simulink model "H175_Stage_01_Anode_Cathode"  (R2023a)
settings: Solver=VariableStepAuto  StartTime=0.0  StopTime=500  RelTol=1e-3
values from neighbouring files (symbols this model uses):
  anode_tube_D = 0.01    [All_Properties.mat]    (also in anode_subsystem_parameters.m; environment_parameters.m)
  D = 0.01    [All_Properties.mat]    (also in anode_subsystem_parameters.m)
  densityHydrogen = 0.0899    [All_Properties.mat]    (also in Valve_Init.m; anode_subsystem_parameters.m)
  Fischer_EMTC120K_supplier_mdot_TLU = [33.385172 57.11265182 82.35238332 173.9183787 230.2050798 50.1655574 86.1774137 122.96585 210.0188714 258.8737112 70.20710678 115.3896052 ... (25 elements, 5x5)]    [All_Properties.mat]    (also in cathode_subsystem_parameters.m = [33.385172 50.1655574 70.20710678 87.4902972 105.3161257)
  Fischer_EMTC120K_supplier_pr_TLU = [2.452176848 3.067593046 4.01020547 5.11549365 6.10066015 2.450765612 3.07166407 4.0616557 5.112468546 6.108742034 2.432340262 3.033516574 ... (25 elements, 5x5)]    [All_Properties.mat]    (also in cathode_subsystem_parameters.m = [2.452176848 2.450765612 2.432340262 2.407245766 2.37067916)
  Kv_VL6112 = 0.8    [All_Properties.mat]    (also in anode_subsystem_parameters.m)
  N2_T = [-56.55 -50 -40 -30 -20 -10 -5 -4 -3 -2 -1 0 ... (52 elements, 1x52)]    [All_Properties.mat]    (also in anode_subsystem_parameters.m = [-56.55 -50 -40 -30 -20 -10 -5 -4 -3 -2 -1 0 1 2 3 4 5 10 20; environment_parameters.m = [-56.55, -50:10:-10, -5:1:5, 10:10:350]; stack_model_harness_parameters.m = [-56.55, -50:10:-10, -5:1:5, 10:10:350])
  p_range = 0.005    [All_Properties.mat]    (also in anode_subsystem_parameters.m)
  r_max = 0.2    [All_Properties.mat]    (also in anode_subsystem_parameters.m)
  r_min = 0.0001    [All_Properties.mat]    (also in anode_subsystem_parameters.m)
  responseTimeValve = 0.013    [All_Properties.mat]    (also in anode_subsystem_parameters.m)
undefined symbols (not defined in the file or in its folder): sigbuilder_block
libraries: fl_lib x168, nesl_utility x116, SimscapeFluids_lib x8, slpidlib x5, simulink x1
(part 6 of 8)

== system H175_Stage_01_Anode_Cathode/Plant Model H175-Cathode-S1/LT-Cooling ==
  Convective Heat Transfer1 : fl_lib/Thermal/Thermal Elements/Convective Heat Transfer  thermal_type=foundation.enum.constant_variable.constant  area=10.8 m^2  heat_tr_coeff=3465 W/(m^2 * K)  min_heat_tr_coeff=1e-3 W/(K*m^2)  T_specify=off  T_priority=None  T=0 K  T_nominal_specify=off  T_nominal_unit=K  T_nominal_value=1  Q_specify=off  Q_priority=None  Q=0 W  Q_nominal_specify=off  Q_nominal_unit=W  Q_nominal_value=1
  Convective Heat Transfer2 : fl_lib/Thermal/Thermal Elements/Convective Heat Transfer  thermal_type=foundation.enum.constant_variable.constant  area=10.8 m^2  heat_tr_coeff=447*4 W/(m^2 * K)  min_heat_tr_coeff=1e-3 W/(K*m^2)  T_specify=off  T_priority=None  T=0 K  T_nominal_specify=off  T_nominal_unit=K  T_nominal_value=1  Q_specify=off  Q_priority=None  Q=0 W  Q_nominal_specify=off  Q_nominal_unit=W  Q_nominal_value=1
  Coolant Tank1 : Subsystem  Tag=PublishSubsystem  mask(Coolant Tank){A=100, x_init=.25}
      mask prompts: A "Tank area (m^2)"; x_init "Initial coolant level (m)"
      mask help: This subsystem models an expansion tank for the coolant system.
  Environment Temperature4 : fl_lib/Thermal/Thermal Sources/Temperature Source  temperature=20 degC
  Glysantin G20 : SimscapeFluids_lib/Thermal Liquid/Utilities/Thermal Liquid Properties (TL)  fluid_list=fluids.thermal_liquid.utilities.enum.thermal_liquid_fluid_list.ethylene_glycol  concentration_param_EG=fluids.thermal_liquid.utilities.enum.thermal_liquid_concentration.volume_fraction  concentration_param_PG=fluids.thermal_liquid.utilities.enum.thermal_liquid_concentration.volume_fraction  c_mass_SW=3.5e-3  c_mass_EG=0.1  c_mass_PG=0.1  c_mass_GL=0.1  c_vol_EG=0.5  c_vol_PG=0.1  beta_const_EG=2.1791 GPa  beta_const_PG=2.1791 GPa  beta_const_GL=2.1791 GPa  p_min_EG=0.01 MPa  p_min_PG=0.01 MPa  p_min_GL=0.01 MPa  p_max_EG=50 MPa  p_max_PG=50 MPa  p_max_GL=50 MPa  p_atm=1 bar  properties_range_check=simscape.enum.assert.action.error
  Pipe (TL)1 : fl_lib/Thermal Liquid/Elements/Pipe (TL)  length=1 m  area=10.8 m^2  Dh=0.1 m  length_add=10 m  roughness=15e-6 m  Re_lam=2000  Re_tur=4000  shape_factor=64  Nu_lam=133.3  dynamic_compressibility=simscape.enum.onoff.on  inertia=simscape.enum.onoff.off  p0=0.101325 MPa  T0=293.15 K  mdot0=0 kg/s
  Pump1 : fl_lib/Thermal Liquid/Sources/Controlled Mass Flow Rate Source (TL)  power_spec=foundation.enum.power_spec.isentropic  area=.002 m^2
      settings: InternalSimscapePortConfiguration="{\"Bottom\":[],\"Left\":[{\"id\":\"A\",\"label\":\"A\",\"type\":\"foundation.thermal_liquid.thermal_liquid\"},{\"id\":\"M\",\"label\":\"M\",\"type\":\"input\"}],\"Right\":[{\"id\":\"B\",\"label\":\"B\",\"type\":\"foundation.thermal_liquid.thermal_liquid\"}],\"Top\":[]}"
  Radiator1 : fl_lib/Thermal Liquid/Elements/Pipe (TL)  length=1 m  area=10.8 m^2  Dh=.1 m  length_add=1 m  roughness=15e-6 m  Re_lam=2000  Re_tur=4000  shape_factor=64  Nu_lam=500  dynamic_compressibility=simscape.enum.onoff.on  inertia=simscape.enum.onoff.off  p0=.103 MPa  T0=20 degC  mdot0=0 kg/s
  Thermal Mass1 : fl_lib/Thermal/Thermal Elements/Thermal Mass  mass_type=foundation.enum.constant_variable.constant  mass=5 kg  sp_heat=447 J/(K*kg)  mass_min=1e-6 kg  num_ports=foundation.enum.numPorts2.two  m_specify=off  m_priority=High  m=1 kg  m_nominal_specify=off  m_nominal_unit=kg  m_nominal_value=1  T_specify=off  T_priority=High  T=300 K  T_nominal_specify=off  T_nominal_unit=K  T_nominal_value=1  Q_specify=off  Q_priority=None  Q=0 W  Q_nominal_specify=off  Q_nominal_unit=W  Q_nominal_value=1
      settings: InternalSimscapePortConfiguration="{\"Bottom\":[],\"Left\":[{\"id\":\"M\",\"label\":\"\",\"type\":\"foundation.thermal.thermal\"}],\"Right\":[{\"id\":\"N\",\"label\":\"\",\"type\":\"foundation.thermal.thermal\"}],\"Top\":[]}"
  Thermal Mass2 : fl_lib/Thermal/Thermal Elements/Thermal Mass  mass_type=foundation.enum.constant_variable.constant  mass=1 kg  sp_heat=910 J/kg/K  mass_min=1e-6 kg  num_ports=foundation.enum.numPorts2.one  m_specify=off  m_priority=High  m=1 kg  m_nominal_specify=off  m_nominal_unit=kg  m_nominal_value=1  T_specify=on  T_priority=High  T=20 degC  T_nominal_specify=off  T_nominal_unit=K  T_nominal_value=1  Q_specify=off  Q_priority=None  Q=0 W  Q_nominal_specify=off  Q_nominal_unit=W  Q_nominal_value=1
  Conn1 : PMIOPort  Side=Left
  Conn2 : PMIOPort  Port=2  Side=Right
  connections:
  Thermal Mass1/RConn1 -- Pipe (TL)1/LConn2
  Radiator1/LConn1 -- Pipe (TL)1/RConn1
  Convective Heat Transfer1/LConn1 -- Radiator1/LConn2
  Pipe (TL)1/LConn1 -- Glysantin G20/RConn1 -- Pump1/RConn1
  Coolant Tank1/RConn1 -- Pump1/LConn1 -- Radiator1/RConn1
  Conn1/RConn1 -- Pump1/LConn2
  Thermal Mass1/LConn1 -- Convective Heat Transfer2/RConn1
  Convective Heat Transfer1/RConn1 -- Thermal Mass2/LConn1 -- Environment Temperature4/LConn1
  Conn2/RConn1 -- Convective Heat Transfer2/LConn1

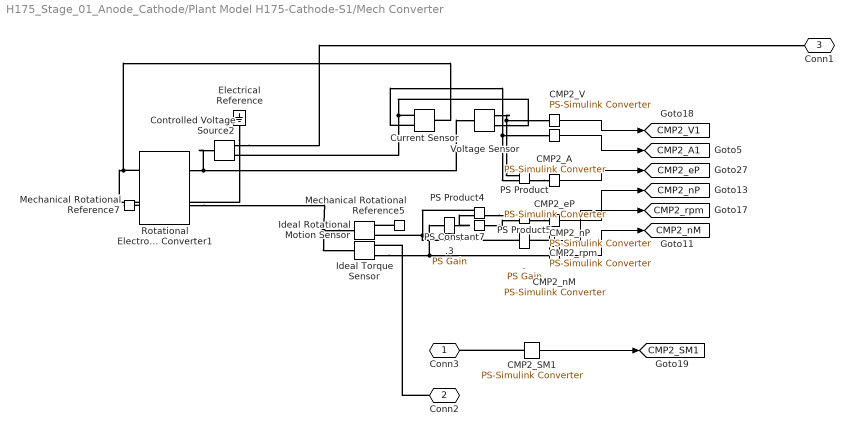
== system H175_Stage_01_Anode_Cathode/Plant Model H175-Cathode-S1/Mech Converter ==
  . : fl_lib/Physical Signals/Functions/PS Gain  gain=1/(0.1047198*1000)
  .3 : fl_lib/Physical Signals/Functions/PS Gain  gain=1/(0.1047198*60)
  CMP2_A : nesl_utility/PS-Simulink Converter  PhysicalDomain=network_engine_domain  SubClassName=ps_output  LeftPortType=input  RightPortType=output  PseudoPeriodic=off  Frequencies=[]  VectorFormat=inherit  Unit=inherit  AffineConversion=off
  CMP2_SM1 : nesl_utility/PS-Simulink Converter  PhysicalDomain=network_engine_domain  SubClassName=ps_output  LeftPortType=input  RightPortType=output  PseudoPeriodic=off  Frequencies=[]  VectorFormat=inherit  Unit=inherit  AffineConversion=off
  CMP2_V : nesl_utility/PS-Simulink Converter  PhysicalDomain=network_engine_domain  SubClassName=ps_output  LeftPortType=input  RightPortType=output  PseudoPeriodic=off  Frequencies=[]  VectorFormat=inherit  Unit=inherit  AffineConversion=off
  CMP2_eP : nesl_utility/PS-Simulink Converter  PhysicalDomain=network_engine_domain  SubClassName=ps_output  LeftPortType=input  RightPortType=output  PseudoPeriodic=off  Frequencies=[]  VectorFormat=inherit  Unit=inherit  AffineConversion=off
  CMP2_nM : nesl_utility/PS-Simulink Converter  PhysicalDomain=network_engine_domain  SubClassName=ps_output  LeftPortType=input  RightPortType=output  PseudoPeriodic=off  Frequencies=[]  VectorFormat=1-D array  Unit=inherit  AffineConversion=off
  CMP2_nP : nesl_utility/PS-Simulink Converter  PhysicalDomain=network_engine_domain  SubClassName=ps_output  LeftPortType=input  RightPortType=output  PseudoPeriodic=off  Frequencies=[]  VectorFormat=inherit  Unit=inherit  AffineConversion=off
  CMP2_rpm : nesl_utility/PS-Simulink Converter  PhysicalDomain=network_engine_domain  SubClassName=ps_output  LeftPortType=input  RightPortType=output  PseudoPeriodic=off  Frequencies=[]  VectorFormat=inherit  Unit=inherit  AffineConversion=off
  Controlled Voltage Source2 : fl_lib/Electrical/Electrical Sources/Controlled Voltage Source
  Current Sensor : fl_lib/Electrical/Electrical Sensors/Current Sensor
  Electrical Reference : fl_lib/Electrical/Electrical Elements/Electrical Reference
  Ideal Rotational Motion Sensor : fl_lib/Mechanical/Mechanical Sensors/Ideal Rotational Motion Sensor  reference=foundation.enum.MeasurementReference.difference  acceleration_port=false  velocity_port=true  position_port=false  wrap_angle=false  offset=0 rad
      settings: InternalSimscapePortConfiguration="{\"Bottom\":[],\"Left\":[{\"id\":\"R\",\"label\":\"R\",\"type\":\"foundation.mechanical.rotational.rotational\"}],\"Right\":[{\"id\":\"C\",\"label\":\"C\",\"type\":\"foundation.mechanical.rotational.rotational\"},{\"id\":\"W\",\"label\":\"W\",\"type\":\"output\"}],\"Top\":[]}"
  Ideal Torque Sensor : fl_lib/Mechanical/Mechanical Sensors/Ideal Torque Sensor
  Mechanical Rotational Reference5 : fl_lib/Mechanical/Rotational Elements/Mechanical Rotational Reference
  Mechanical Rotational Reference7 : fl_lib/Mechanical/Rotational Elements/Mechanical Rotational Reference
  PS Constant7 : fl_lib/Physical Signals/Sources/PS Constant  constant=2*pi
  PS Product : fl_lib/Physical Signals/Functions/PS Product
  PS Product4 : fl_lib/Physical Signals/Functions/PS Product
  PS Product5 : fl_lib/Physical Signals/Functions/PS Product
  Rotational Electromechanical Converter1 : fl_lib/Electrical/Electrical Elements/Rotational Electromechanical Converter  K=0.00409090909090909090909090909091 V/rpm  i_specify=off  i_priority=None  i=0 A  i_nominal_specify=off  i_nominal_unit=A  i_nominal_value=1  v_specify=off  v_priority=None  v=50 V  v_nominal_specify=off  v_nominal_unit=V  v_nominal_value=1  t_specify=off  t_priority=None  t=0 N*m  t_nominal_specify=off  t_nominal_unit=N*m  t_nominal_value=1  w_specify=off  w_priority=None  w=0 rad/s  w_nominal_specify=off  w_nominal_unit=rad/s  w_nominal_value=1
  Voltage Sensor : fl_lib/Electrical/Electrical Sensors/Voltage Sensor
  Conn3 : PMIOPort  Side=Left
  Conn2 : PMIOPort  Port=2  Side=Left
  Conn1 : PMIOPort  Port=3  Side=Right
  tag scope: CMP2_A1=global, CMP2_SM1=global, CMP2_V1=global, CMP2_eP=global, CMP2_nM=global, CMP2_nP=global, CMP2_rpm=global
  wires:
  CMP2_eP/1 -> [CMP2_eP]
  CMP2_V/1 -> [CMP2_V1]
  CMP2_A/1 -> [CMP2_A1]
  CMP2_nM/1 -> [CMP2_nM]
  CMP2_rpm/1 -> [CMP2_rpm]
  CMP2_nP/1 -> [CMP2_nP]
  CMP2_SM1/1 -> [CMP2_SM1]
  connections:
  CMP2_rpm/LConn1 -- ./RConn1
  PS Constant7/RConn1 -- PS Product5/LConn2
  Rotational Electromechanical Converter1/RConn2 -- Mechanical Rotational Reference7/LConn1
  Controlled Voltage Source2/LConn1 -- Voltage Sensor/LConn1 -- Rotational Electromechanical Converter1/LConn1
  Electrical Reference/LConn1 -- Current Sensor/LConn1 -- Rotational Electromechanical Converter1/RConn1
  Current Sensor/RConn1 -- PS Product/LConn1 -- CMP2_A/LConn1
  Controlled Voltage Source2/RConn1 -- Conn1/RConn1
  Ideal Rotational Motion Sensor/LConn1 -- Rotational Electromechanical Converter1/LConn2 -- Ideal Torque Sensor/LConn1
  Current Sensor/RConn2 -- Voltage Sensor/RConn2 -- Controlled Voltage Source2/RConn2
  PS Product/RConn1 -- CMP2_eP/LConn1
  .3/RConn1 -- PS Product4/LConn2
  PS Product4/RConn1 -- PS Product5/LConn1
  Ideal Torque Sensor/RConn2 -- CMP2_nM/LConn1 -- .3/LConn1
  PS Product5/RConn1 -- CMP2_nP/LConn1
  Voltage Sensor/RConn1 -- PS Product/LConn2 -- CMP2_V/LConn1
  ./LConn1 -- PS Product4/LConn1 -- Ideal Rotational Motion Sensor/RConn2
  Mechanical Rotational Reference5/LConn1 -- Ideal Rotational Motion Sensor/RConn1
  Conn2/RConn1 -- Ideal Torque Sensor/RConn1
  CMP2_SM1/LConn1 -- Conn3/RConn1

== system H175_Stage_01_Anode_Cathode/Plant Model H175-Cathode-S1/S1 ==
  Absolute Reference (G) : fl_lib/Gas/Elements/Absolute Reference (G)
      settings: InternalSimscapePortConfiguration="{\"Bottom\":[],\"Left\":[{\"id\":\"A\",\"label\":\"\",\"type\":\"foundation.gas.gas\"}],\"Right\":[],\"Top\":[]}"
  Bus Creator : BusCreator  Inputs=3
  Mass & Energy Flow Rate Sensor (G) : fl_lib/Gas/Sensors/Flow Rate Sensor (G)  mass_flow_measure=true  volumetric_flow_measure=false  volumetric_flow_conditions=foundation.enum.volumetric_flow_conditions.actual  p_std=0.101325 MPa  T_std=20 degC  energy_flow_measure=true
      settings: InternalSimscapePortConfiguration="{\"Bottom\":[{\"id\":\"PHI\",\"label\":\"φ\",\"type\":\"output\"}],\"Left\":[{\"id\":\"A\",\"label\":\"A\",\"type\":\"foundation.gas.gas\"}],\"Right\":[{\"id\":\"B\",\"label\":\"B\",\"type\":\"foundation.gas.gas\"},{\"id\":\"M\",\"label\":\"M\",\"type\":\"output\"}],\"Top\":[]}"
  Pressure & Temperature Sensor (G)4 : fl_lib/Gas/Sensors/Pressure & Temperature Sensor (G)  reference=foundation.enum.MeasurementReference.difference  pressure=true  pressure_spec=foundation.enum.PressureMeasementSpec.Absolute  temperature=true
      settings: InternalSimscapePortConfiguration="{\"Bottom\":[{\"id\":\"T\",\"label\":\"T\",\"type\":\"output\"}],\"Left\":[{\"id\":\"A\",\"label\":\"A\",\"type\":\"foundation.gas.gas\"}],\"Right\":[{\"id\":\"B\",\"label\":\"B\",\"type\":\"foundation.gas.gas\"},{\"id\":\"P\",\"label\":\"P\",\"type\":\"output\"}],\"Top\":[]}"
  aPres_S1 : nesl_utility/PS-Simulink Converter  PhysicalDomain=network_engine_domain  SubClassName=ps_output  LeftPortType=input  RightPortType=output  PseudoPeriodic=off  Frequencies=[]  VectorFormat=inherit  Unit=inherit  AffineConversion=off
  aTemp_S1 : nesl_utility/PS-Simulink Converter  PhysicalDomain=network_engine_domain  SubClassName=ps_output  LeftPortType=input  RightPortType=output  PseudoPeriodic=off  Frequencies=[]  VectorFormat=inherit  Unit=degC  AffineConversion=off
  aTemp_S2 : nesl_utility/PS-Simulink Converter  PhysicalDomain=network_engine_domain  SubClassName=ps_output  LeftPortType=input  RightPortType=output  PseudoPeriodic=off  Frequencies=[]  VectorFormat=inherit  Unit=inherit  AffineConversion=off
  Conn1 : PMIOPort  Side=Left
  Conn2 : PMIOPort  Port=2  Side=Right
  tag scope: S1=global
  wires:
  aTemp_S1/1 -> Bus Creator/2  "aTemp_S1"
  aPres_S1/1 -> Bus Creator/1  "aPres_S1"
  aTemp_S2/1 -> Bus Creator/3  "mFlow_S1"
  Bus Creator/1 -> [S1]
  connections:
  Absolute Reference (G)/LConn1 -- Pressure & Temperature Sensor (G)4/RConn1
  aPres_S1/LConn1 -- Pressure & Temperature Sensor (G)4/RConn2
  aTemp_S1/LConn1 -- Pressure & Temperature Sensor (G)4/RConn3
  Pressure & Temperature Sensor (G)4/LConn1 -- Mass & Energy Flow Rate Sensor (G)/LConn1 -- Conn1/RConn1
  Mass & Energy Flow Rate Sensor (G)/RConn2 -- aTemp_S2/LConn1
  Mass & Energy Flow Rate Sensor (G)/RConn1 -- Conn2/RConn1

== system H175_Stage_01_Anode_Cathode/Plant Model H175-Cathode-S1/S2 ==
  Absolute Reference (G) : fl_lib/Gas/Elements/Absolute Reference (G)
      settings: InternalSimscapePortConfiguration="{\"Bottom\":[],\"Left\":[{\"id\":\"A\",\"label\":\"\",\"type\":\"foundation.gas.gas\"}],\"Right\":[],\"Top\":[]}"
  Bus Creator : BusCreator  Inputs=3
  Mass & Energy Flow Rate Sensor (G) : fl_lib/Gas/Sensors/Flow Rate Sensor (G)  mass_flow_measure=true  volumetric_flow_measure=false  volumetric_flow_conditions=foundation.enum.volumetric_flow_conditions.actual  p_std=0.101325 MPa  T_std=20 degC  energy_flow_measure=true
      settings: InternalSimscapePortConfiguration="{\"Bottom\":[{\"id\":\"PHI\",\"label\":\"φ\",\"type\":\"output\"}],\"Left\":[{\"id\":\"A\",\"label\":\"A\",\"type\":\"foundation.gas.gas\"}],\"Right\":[{\"id\":\"B\",\"label\":\"B\",\"type\":\"foundation.gas.gas\"},{\"id\":\"M\",\"label\":\"M\",\"type\":\"output\"}],\"Top\":[]}"
  Pressure & Temperature Sensor (G)4 : fl_lib/Gas/Sensors/Pressure & Temperature Sensor (G)  reference=foundation.enum.MeasurementReference.difference  pressure=true  pressure_spec=foundation.enum.PressureMeasementSpec.Absolute  temperature=true
      settings: InternalSimscapePortConfiguration="{\"Bottom\":[{\"id\":\"T\",\"label\":\"T\",\"type\":\"output\"}],\"Left\":[{\"id\":\"A\",\"label\":\"A\",\"type\":\"foundation.gas.gas\"}],\"Right\":[{\"id\":\"B\",\"label\":\"B\",\"type\":\"foundation.gas.gas\"},{\"id\":\"P\",\"label\":\"P\",\"type\":\"output\"}],\"Top\":[]}"
  To Workspace : ToWorkspace  VariableName=EAC_aPres_S2  SaveFormat=Timeseries  SampleTime=-1
  aPres_S1 : nesl_utility/PS-Simulink Converter  PhysicalDomain=network_engine_domain  SubClassName=ps_output  LeftPortType=input  RightPortType=output  PseudoPeriodic=off  Frequencies=[]  VectorFormat=inherit  Unit=inherit  AffineConversion=off
  aTemp_S1 : nesl_utility/PS-Simulink Converter  PhysicalDomain=network_engine_domain  SubClassName=ps_output  LeftPortType=input  RightPortType=output  PseudoPeriodic=off  Frequencies=[]  VectorFormat=inherit  Unit=degC  AffineConversion=off
  mFlow_S2 : nesl_utility/PS-Simulink Converter  PhysicalDomain=network_engine_domain  SubClassName=ps_output  LeftPortType=input  RightPortType=output  PseudoPeriodic=off  Frequencies=[]  VectorFormat=inherit  Unit=kg/s  AffineConversion=off
  Conn1 : PMIOPort  Side=Left
  Conn2 : PMIOPort  Port=2  Side=Right
  tag scope: S2=global
  wires:
  aPres_S1/1 -> To Workspace/1, Bus Creator/1  "aPres_S2"
  aTemp_S1/1 -> Bus Creator/2  "aTemp_S2"
  mFlow_S2/1 -> Bus Creator/3  "mFlow_S2"
  Bus Creator/1 -> [S2]
  connections:
  Pressure & Temperature Sensor (G)4/LConn1 -- Mass & Energy Flow Rate Sensor (G)/LConn1 -- Conn1/RConn1
  Absolute Reference (G)/LConn1 -- Pressure & Temperature Sensor (G)4/RConn1
  aPres_S1/LConn1 -- Pressure & Temperature Sensor (G)4/RConn2
  aTemp_S1/LConn1 -- Pressure & Temperature Sensor (G)4/RConn3
  Mass & Energy Flow Rate Sensor (G)/RConn1 -- Conn2/RConn1
  Mass & Energy Flow Rate Sensor (G)/RConn2 -- mFlow_S2/LConn1

== system H175_Stage_01_Anode_Cathode/Plant Model H175-Cathode-S1/S3 ==
  Absolute Reference (MA) : fl_lib/Moist Air/Elements/Absolute Reference (MA)
  Bus Creator : BusCreator  Inputs=9
  Humidity & Trace Gas Sensor (MA)1 : fl_lib/Moist Air/Sensors/Humidity & Trace Gas Sensor (MA)  moisture_on=true  moisture_spec=foundation.enum.moisture_spec.relative_humidity  trace_gas_on=true  trace_gas_spec=foundation.enum.trace_gas_spec.mass_fraction
      settings: InternalSimscapePortConfiguration="{\"Bottom\":[],\"Left\":[{\"id\":\"A\",\"label\":\"A\",\"type\":\"foundation.moist_air.moist_air\"}],\"Right\":[{\"id\":\"W\",\"label\":\"W\",\"type\":\"output\"},{\"id\":\"G\",\"label\":\"G\",\"type\":\"output\"}],\"Top\":[]}"
  Mass & Energy Flow Rate Sensor (MA) : fl_lib/Moist Air/Sensors/Flow Rate Sensor (MA)  mass_flow_measure=true  volumetric_flow_measure=false  volumetric_flow_conditions=foundation.enum.volumetric_flow_conditions.actual  p_std=0.101325 MPa  T_std=20 degC  RH_std=0.65  energy_flow_measure=true  vapor_flow_measure=true  gas_flow_measure=true
      settings: InternalSimscapePortConfiguration="{\"Bottom\":[{\"id\":\"PHI\",\"label\":\"φ\",\"type\":\"output\"}],\"Left\":[{\"id\":\"A\",\"label\":\"A\",\"type\":\"foundation.moist_air.moist_air\"},{\"id\":\"Mw\",\"label\":\"Mw\",\"type\":\"output\"},{\"id\":\"Mg\",\"label\":\"Mg\",\"type\":\"output\"}],\"Right\":[{\"id\":\"B\",\"label\":\"B\",\"type\":\"foundation.moist_air.moist_air\"},{\"id\":\"M\",\"label\":\"M\",\"type\":\"output\"}],\"Top\":[]}"
  MixDensity : nesl_utility/PS-Simulink Converter  PhysicalDomain=network_engine_domain  SubClassName=ps_output  LeftPortType=input  RightPortType=output  PseudoPeriodic=off  Frequencies=[]  VectorFormat=inherit  Unit=inherit  AffineConversion=off
  MixSEnthaply : nesl_utility/PS-Simulink Converter  PhysicalDomain=network_engine_domain  SubClassName=ps_output  LeftPortType=input  RightPortType=output  PseudoPeriodic=off  Frequencies=[]  VectorFormat=inherit  Unit=inherit  AffineConversion=off
  Pressure & Temperature Sensor (MA) : fl_lib/Moist Air/Sensors/Pressure & Temperature Sensor (MA)  reference=foundation.enum.MeasurementReference.difference  pressure=true  pressure_spec=foundation.enum.PressureMeasementSpec.Absolute  temperature=true
      settings: InternalSimscapePortConfiguration="{\"Bottom\":[{\"id\":\"T\",\"label\":\"T\",\"type\":\"output\"}],\"Left\":[{\"id\":\"A\",\"label\":\"A\",\"type\":\"foundation.moist_air.moist_air\"}],\"Right\":[{\"id\":\"B\",\"label\":\"B\",\"type\":\"foundation.moist_air.moist_air\"},{\"id\":\"P\",\"label\":\"P\",\"type\":\"output\"}],\"Top\":[]}"
  SEntropy : nesl_utility/PS-Simulink Converter  PhysicalDomain=network_engine_domain  SubClassName=ps_output  LeftPortType=input  RightPortType=output  PseudoPeriodic=off  Frequencies=[]  VectorFormat=inherit  Unit=inherit  AffineConversion=off
  SHeat : nesl_utility/PS-Simulink Converter  PhysicalDomain=network_engine_domain  SubClassName=ps_output  LeftPortType=input  RightPortType=output  PseudoPeriodic=off  Frequencies=[]  VectorFormat=inherit  Unit=inherit  AffineConversion=off
  Thermodynamic Properties Sensor (MA) : fl_lib/Moist Air/Sensors/Thermodynamic Properties Sensor (MA)  measurement_mass_spec=foundation.enum.measurement_mass_spec.mixture  enthalpy=true  density=true  specific_heat=true  entropy=true
      settings: InternalSimscapePortConfiguration="{\"Bottom\":[{\"id\":\"CP\",\"label\":\"cp\",\"type\":\"output\"},{\"id\":\"S\",\"label\":\"s\",\"type\":\"output\"}],\"Left\":[{\"id\":\"A\",\"label\":\"A\",\"type\":\"foundation.moist_air.moist_air\"}],\"Right\":[{\"id\":\"H\",\"label\":\"h\",\"type\":\"output\"},{\"id\":\"RHO\",\"label\":\"ρ\",\"type\":\"output\"}],\"Top\":[]}"
  aPres_S4 : nesl_utility/PS-Simulink Converter  PhysicalDomain=network_engine_domain  SubClassName=ps_output  LeftPortType=input  RightPortType=output  PseudoPeriodic=off  Frequencies=[]  VectorFormat=inherit  Unit=inherit  AffineConversion=off
  aTemp : nesl_utility/PS-Simulink Converter  PhysicalDomain=network_engine_domain  SubClassName=ps_output  LeftPortType=input  RightPortType=output  PseudoPeriodic=off  Frequencies=[]  VectorFormat=inherit  Unit=inherit  AffineConversion=off
  mFlow : nesl_utility/PS-Simulink Converter  PhysicalDomain=network_engine_domain  SubClassName=ps_output  LeftPortType=input  RightPortType=output  PseudoPeriodic=off  Frequencies=[]  VectorFormat=inherit  Unit=inherit  AffineConversion=off
  mFraction : nesl_utility/PS-Simulink Converter  PhysicalDomain=network_engine_domain  SubClassName=ps_output  LeftPortType=input  RightPortType=output  PseudoPeriodic=off  Frequencies=[]  VectorFormat=inherit  Unit=inherit  AffineConversion=off
  relHum : nesl_utility/PS-Simulink Converter  PhysicalDomain=network_engine_domain  SubClassName=ps_output  LeftPortType=input  RightPortType=output  PseudoPeriodic=off  Frequencies=[]  VectorFormat=inherit  Unit=inherit  AffineConversion=off
  Conn2 : PMIOPort  Side=Left
  Conn1 : PMIOPort  Port=2  Side=Right
  tag scope: S3=global
  wires:
  aTemp/1 -> Bus Creator/2  "aTemp_S3"
  aPres_S4/1 -> Bus Creator/1  "aPres_S3"
  SEntropy/1 -> Bus Creator/9  "SEntropy_S3"
  MixSEnthaply/1 -> Bus Creator/6  "MixSEnthalpy_S3"
  MixDensity/1 -> Bus Creator/7  "MixDensity_S3"
  mFraction/1 -> Bus Creator/5  "mFraction_S3"
  mFlow/1 -> Bus Creator/3  "mFlow_S3"
  relHum/1 -> Bus Creator/4  "relHum_S3"
  SHeat/1 -> Bus Creator/8  "SHeat_S3"
  Bus Creator/1 -> [S3]
  connections:
  Mass & Energy Flow Rate Sensor (MA)/LConn1 -- Conn1/RConn1
  Humidity & Trace Gas Sensor (MA)1/RConn1 -- relHum/LConn1
  MixSEnthaply/LConn1 -- Thermodynamic Properties Sensor (MA)/RConn1
  MixDensity/LConn1 -- Thermodynamic Properties Sensor (MA)/RConn2
  SHeat/LConn1 -- Thermodynamic Properties Sensor (MA)/RConn4
  aTemp/LConn1 -- Pressure & Temperature Sensor (MA)/RConn3
  SEntropy/LConn1 -- Thermodynamic Properties Sensor (MA)/RConn3
  Conn2/RConn1 -- Mass & Energy Flow Rate Sensor (MA)/RConn1 -- Thermodynamic Properties Sensor (MA)/LConn1 -- Pressure & Temperature Sensor (MA)/LConn1 -- Humidity & Trace Gas Sensor (MA)1/LConn1
  mFlow/LConn1 -- Mass & Energy Flow Rate Sensor (MA)/RConn2
  Pressure & Temperature Sensor (MA)/RConn2 -- aPres_S4/LConn1
  Humidity & Trace Gas Sensor (MA)1/RConn2 -- mFraction/LConn1
  Absolute Reference (MA)/LConn1 -- Pressure & Temperature Sensor (MA)/RConn1

== system H175_Stage_01_Anode_Cathode/Plant Model H175-Cathode-S1/S4 ==
  Absolute Reference (MA) : fl_lib/Moist Air/Elements/Absolute Reference (MA)
  Bus Creator : BusCreator  Inputs=9
  Humidity & Trace Gas Sensor (MA)1 : fl_lib/Moist Air/Sensors/Humidity & Trace Gas Sensor (MA)  moisture_on=true  moisture_spec=foundation.enum.moisture_spec.relative_humidity  trace_gas_on=true  trace_gas_spec=foundation.enum.trace_gas_spec.mass_fraction
      settings: InternalSimscapePortConfiguration="{\"Bottom\":[],\"Left\":[{\"id\":\"A\",\"label\":\"A\",\"type\":\"foundation.moist_air.moist_air\"}],\"Right\":[{\"id\":\"W\",\"label\":\"W\",\"type\":\"output\"},{\"id\":\"G\",\"label\":\"G\",\"type\":\"output\"}],\"Top\":[]}"
  Mass & Energy Flow Rate Sensor (MA) : fl_lib/Moist Air/Sensors/Flow Rate Sensor (MA)  mass_flow_measure=true  volumetric_flow_measure=false  volumetric_flow_conditions=foundation.enum.volumetric_flow_conditions.actual  p_std=0.101325 MPa  T_std=20 degC  RH_std=0.65  energy_flow_measure=true  vapor_flow_measure=true  gas_flow_measure=true
      settings: InternalSimscapePortConfiguration="{\"Bottom\":[{\"id\":\"PHI\",\"label\":\"φ\",\"type\":\"output\"}],\"Left\":[{\"id\":\"A\",\"label\":\"A\",\"type\":\"foundation.moist_air.moist_air\"},{\"id\":\"Mw\",\"label\":\"Mw\",\"type\":\"output\"},{\"id\":\"Mg\",\"label\":\"Mg\",\"type\":\"output\"}],\"Right\":[{\"id\":\"B\",\"label\":\"B\",\"type\":\"foundation.moist_air.moist_air\"},{\"id\":\"M\",\"label\":\"M\",\"type\":\"output\"}],\"Top\":[]}"
  MixDensity : nesl_utility/PS-Simulink Converter  PhysicalDomain=network_engine_domain  SubClassName=ps_output  LeftPortType=input  RightPortType=output  PseudoPeriodic=off  Frequencies=[]  VectorFormat=inherit  Unit=inherit  AffineConversion=off
  MixSEnthaply : nesl_utility/PS-Simulink Converter  PhysicalDomain=network_engine_domain  SubClassName=ps_output  LeftPortType=input  RightPortType=output  PseudoPeriodic=off  Frequencies=[]  VectorFormat=inherit  Unit=inherit  AffineConversion=off
  Pressure & Temperature Sensor (MA) : fl_lib/Moist Air/Sensors/Pressure & Temperature Sensor (MA)  reference=foundation.enum.MeasurementReference.difference  pressure=true  pressure_spec=foundation.enum.PressureMeasementSpec.Absolute  temperature=true
      settings: InternalSimscapePortConfiguration="{\"Bottom\":[{\"id\":\"T\",\"label\":\"T\",\"type\":\"output\"}],\"Left\":[{\"id\":\"A\",\"label\":\"A\",\"type\":\"foundation.moist_air.moist_air\"}],\"Right\":[{\"id\":\"B\",\"label\":\"B\",\"type\":\"foundation.moist_air.moist_air\"},{\"id\":\"P\",\"label\":\"P\",\"type\":\"output\"}],\"Top\":[]}"
  SEntropy : nesl_utility/PS-Simulink Converter  PhysicalDomain=network_engine_domain  SubClassName=ps_output  LeftPortType=input  RightPortType=output  PseudoPeriodic=off  Frequencies=[]  VectorFormat=inherit  Unit=inherit  AffineConversion=off
  SHeat : nesl_utility/PS-Simulink Converter  PhysicalDomain=network_engine_domain  SubClassName=ps_output  LeftPortType=input  RightPortType=output  PseudoPeriodic=off  Frequencies=[]  VectorFormat=inherit  Unit=inherit  AffineConversion=off
  Thermodynamic Properties Sensor (MA) : fl_lib/Moist Air/Sensors/Thermodynamic Properties Sensor (MA)  measurement_mass_spec=foundation.enum.measurement_mass_spec.mixture  enthalpy=true  density=true  specific_heat=true  entropy=true
      settings: InternalSimscapePortConfiguration="{\"Bottom\":[{\"id\":\"CP\",\"label\":\"cp\",\"type\":\"output\"},{\"id\":\"S\",\"label\":\"s\",\"type\":\"output\"}],\"Left\":[{\"id\":\"A\",\"label\":\"A\",\"type\":\"foundation.moist_air.moist_air\"}],\"Right\":[{\"id\":\"H\",\"label\":\"h\",\"type\":\"output\"},{\"id\":\"RHO\",\"label\":\"ρ\",\"type\":\"output\"}],\"Top\":[]}"
  aPres_S4 : nesl_utility/PS-Simulink Converter  PhysicalDomain=network_engine_domain  SubClassName=ps_output  LeftPortType=input  RightPortType=output  PseudoPeriodic=off  Frequencies=[]  VectorFormat=inherit  Unit=inherit  AffineConversion=off
  aTemp : nesl_utility/PS-Simulink Converter  PhysicalDomain=network_engine_domain  SubClassName=ps_output  LeftPortType=input  RightPortType=output  PseudoPeriodic=off  Frequencies=[]  VectorFormat=inherit  Unit=inherit  AffineConversion=off
  mFlow : nesl_utility/PS-Simulink Converter  PhysicalDomain=network_engine_domain  SubClassName=ps_output  LeftPortType=input  RightPortType=output  PseudoPeriodic=off  Frequencies=[]  VectorFormat=inherit  Unit=inherit  AffineConversion=off
  mFraction : nesl_utility/PS-Simulink Converter  PhysicalDomain=network_engine_domain  SubClassName=ps_output  LeftPortType=input  RightPortType=output  PseudoPeriodic=off  Frequencies=[]  VectorFormat=inherit  Unit=inherit  AffineConversion=off
  relHum : nesl_utility/PS-Simulink Converter  PhysicalDomain=network_engine_domain  SubClassName=ps_output  LeftPortType=input  RightPortType=output  PseudoPeriodic=off  Frequencies=[]  VectorFormat=inherit  Unit=inherit  AffineConversion=off
  Conn1 : PMIOPort  Side=Left
  Conn2 : PMIOPort  Port=2  Side=Right
  tag scope: S4=global
  wires:
  SHeat/1 -> Bus Creator/8  "SHeat_S4"
  relHum/1 -> Bus Creator/4  "relHum_S4"
  mFlow/1 -> Bus Creator/3  "mFlow_S4"
  mFraction/1 -> Bus Creator/5  "mFraction_S4"
  MixDensity/1 -> Bus Creator/7  "MixDensity_S4"
  MixSEnthaply/1 -> Bus Creator/6  "MixSEnthalpy_S4"
  SEntropy/1 -> Bus Creator/9  "SEntropy_S4"
  aPres_S4/1 -> Bus Creator/1  "aPres_S4"
  aTemp/1 -> Bus Creator/2  "aTemp_S4"
  Bus Creator/1 -> [S4]
  connections:
  Humidity & Trace Gas Sensor (MA)1/RConn2 -- mFraction/LConn1
  Pressure & Temperature Sensor (MA)/RConn2 -- aPres_S4/LConn1
  Mass & Energy Flow Rate Sensor (MA)/RConn2 -- mFlow/LConn1
  Pressure & Temperature Sensor (MA)/LConn1 -- Thermodynamic Properties Sensor (MA)/LConn1 -- Mass & Energy Flow Rate Sensor (MA)/RConn1 -- Conn2/RConn1 -- Humidity & Trace Gas Sensor (MA)1/LConn1
  SEntropy/LConn1 -- Thermodynamic Properties Sensor (MA)/RConn3
  aTemp/LConn1 -- Pressure & Temperature Sensor (MA)/RConn3
  SHeat/LConn1 -- Thermodynamic Properties Sensor (MA)/RConn4
  MixDensity/LConn1 -- Thermodynamic Properties Sensor (MA)/RConn2
  MixSEnthaply/LConn1 -- Thermodynamic Properties Sensor (MA)/RConn1
  Humidity & Trace Gas Sensor (MA)1/RConn1 -- relHum/LConn1
  Conn1/RConn1 -- Mass & Energy Flow Rate Sensor (MA)/LConn1
  Pressure & Temperature Sensor (MA)/RConn1 -- Absolute Reference (MA)/LConn1

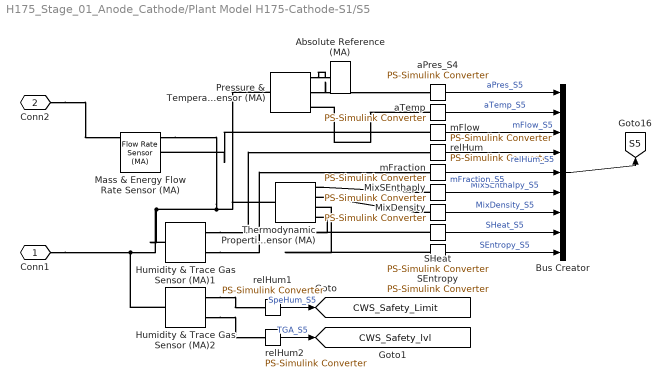
== system H175_Stage_01_Anode_Cathode/Plant Model H175-Cathode-S1/S5 ==
  Absolute Reference (MA) : fl_lib/Moist Air/Elements/Absolute Reference (MA)
  Bus Creator : BusCreator  Inputs=9
  Humidity & Trace Gas Sensor (MA)1 : fl_lib/Moist Air/Sensors/Humidity & Trace Gas Sensor (MA)  moisture_on=true  moisture_spec=foundation.enum.moisture_spec.relative_humidity  trace_gas_on=true  trace_gas_spec=foundation.enum.trace_gas_spec.mass_fraction
      settings: InternalSimscapePortConfiguration="{\"Bottom\":[],\"Left\":[{\"id\":\"A\",\"label\":\"A\",\"type\":\"foundation.moist_air.moist_air\"}],\"Right\":[{\"id\":\"W\",\"label\":\"W\",\"type\":\"output\"},{\"id\":\"G\",\"label\":\"G\",\"type\":\"output\"}],\"Top\":[]}"
  Humidity & Trace Gas Sensor (MA)2 : fl_lib/Moist Air/Sensors/Humidity & Trace Gas Sensor (MA)  moisture_on=true  moisture_spec=foundation.enum.moistureSpec.SpecificHumidity  trace_gas_on=true  trace_gas_spec=foundation.enum.trace_gas_spec.mass_fraction
      settings: InternalSimscapePortConfiguration="{\"Bottom\":[],\"Left\":[{\"id\":\"A\",\"label\":\"A\",\"type\":\"foundation.moist_air.moist_air\"}],\"Right\":[{\"id\":\"W\",\"label\":\"W\",\"type\":\"output\"},{\"id\":\"G\",\"label\":\"G\",\"type\":\"output\"}],\"Top\":[]}"
  Mass & Energy Flow Rate Sensor (MA) : fl_lib/Moist Air/Sensors/Flow Rate Sensor (MA)  mass_flow_measure=true  volumetric_flow_measure=false  volumetric_flow_conditions=foundation.enum.volumetric_flow_conditions.actual  p_std=0.101325 MPa  T_std=20 degC  RH_std=0.65  energy_flow_measure=true  vapor_flow_measure=true  gas_flow_measure=true
      settings: InternalSimscapePortConfiguration="{\"Bottom\":[{\"id\":\"PHI\",\"label\":\"φ\",\"type\":\"output\"}],\"Left\":[{\"id\":\"A\",\"label\":\"A\",\"type\":\"foundation.moist_air.moist_air\"},{\"id\":\"Mw\",\"label\":\"Mw\",\"type\":\"output\"},{\"id\":\"Mg\",\"label\":\"Mg\",\"type\":\"output\"}],\"Right\":[{\"id\":\"B\",\"label\":\"B\",\"type\":\"foundation.moist_air.moist_air\"},{\"id\":\"M\",\"label\":\"M\",\"type\":\"output\"}],\"Top\":[]}"
  MixDensity : nesl_utility/PS-Simulink Converter  PhysicalDomain=network_engine_domain  SubClassName=ps_output  LeftPortType=input  RightPortType=output  PseudoPeriodic=off  Frequencies=[]  VectorFormat=inherit  Unit=inherit  AffineConversion=off
  MixSEnthaply : nesl_utility/PS-Simulink Converter  PhysicalDomain=network_engine_domain  SubClassName=ps_output  LeftPortType=input  RightPortType=output  PseudoPeriodic=off  Frequencies=[]  VectorFormat=inherit  Unit=inherit  AffineConversion=off
  Pressure & Temperature Sensor (MA) : fl_lib/Moist Air/Sensors/Pressure & Temperature Sensor (MA)  reference=foundation.enum.MeasurementReference.difference  pressure=true  pressure_spec=foundation.enum.PressureMeasementSpec.Absolute  temperature=true
      settings: InternalSimscapePortConfiguration="{\"Bottom\":[{\"id\":\"T\",\"label\":\"T\",\"type\":\"output\"}],\"Left\":[{\"id\":\"A\",\"label\":\"A\",\"type\":\"foundation.moist_air.moist_air\"}],\"Right\":[{\"id\":\"B\",\"label\":\"B\",\"type\":\"foundation.moist_air.moist_air\"},{\"id\":\"P\",\"label\":\"P\",\"type\":\"output\"}],\"Top\":[]}"
  SEntropy : nesl_utility/PS-Simulink Converter  PhysicalDomain=network_engine_domain  SubClassName=ps_output  LeftPortType=input  RightPortType=output  PseudoPeriodic=off  Frequencies=[]  VectorFormat=inherit  Unit=inherit  AffineConversion=off
  SHeat : nesl_utility/PS-Simulink Converter  PhysicalDomain=network_engine_domain  SubClassName=ps_output  LeftPortType=input  RightPortType=output  PseudoPeriodic=off  Frequencies=[]  VectorFormat=inherit  Unit=inherit  AffineConversion=off
  Thermodynamic Properties Sensor (MA) : fl_lib/Moist Air/Sensors/Thermodynamic Properties Sensor (MA)  measurement_mass_spec=foundation.enum.measurement_mass_spec.mixture  enthalpy=true  density=true  specific_heat=true  entropy=true
      settings: InternalSimscapePortConfiguration="{\"Bottom\":[{\"id\":\"CP\",\"label\":\"cp\",\"type\":\"output\"},{\"id\":\"S\",\"label\":\"s\",\"type\":\"output\"}],\"Left\":[{\"id\":\"A\",\"label\":\"A\",\"type\":\"foundation.moist_air.moist_air\"}],\"Right\":[{\"id\":\"H\",\"label\":\"h\",\"type\":\"output\"},{\"id\":\"RHO\",\"label\":\"ρ\",\"type\":\"output\"}],\"Top\":[]}"
  aPres_S4 : nesl_utility/PS-Simulink Converter  PhysicalDomain=network_engine_domain  SubClassName=ps_output  LeftPortType=input  RightPortType=output  PseudoPeriodic=off  Frequencies=[]  VectorFormat=inherit  Unit=inherit  AffineConversion=off
  aTemp : nesl_utility/PS-Simulink Converter  PhysicalDomain=network_engine_domain  SubClassName=ps_output  LeftPortType=input  RightPortType=output  PseudoPeriodic=off  Frequencies=[]  VectorFormat=inherit  Unit=inherit  AffineConversion=off
  mFlow : nesl_utility/PS-Simulink Converter  PhysicalDomain=network_engine_domain  SubClassName=ps_output  LeftPortType=input  RightPortType=output  PseudoPeriodic=off  Frequencies=[]  VectorFormat=inherit  Unit=inherit  AffineConversion=off
  mFraction : nesl_utility/PS-Simulink Converter  PhysicalDomain=network_engine_domain  SubClassName=ps_output  LeftPortType=input  RightPortType=output  PseudoPeriodic=off  Frequencies=[]  VectorFormat=inherit  Unit=inherit  AffineConversion=off
  relHum : nesl_utility/PS-Simulink Converter  PhysicalDomain=network_engine_domain  SubClassName=ps_output  LeftPortType=input  RightPortType=output  PseudoPeriodic=off  Frequencies=[]  VectorFormat=inherit  Unit=inherit  AffineConversion=off
  relHum1 : nesl_utility/PS-Simulink Converter  PhysicalDomain=network_engine_domain  SubClassName=ps_output  LeftPortType=input  RightPortType=output  PseudoPeriodic=off  Frequencies=[]  VectorFormat=inherit  Unit=inherit  AffineConversion=off
  relHum2 : nesl_utility/PS-Simulink Converter  PhysicalDomain=network_engine_domain  SubClassName=ps_output  LeftPortType=input  RightPortType=output  PseudoPeriodic=off  Frequencies=[]  VectorFormat=inherit  Unit=inherit  AffineConversion=off
  Conn1 : PMIOPort  Side=Left
  Conn2 : PMIOPort  Port=2  Side=Right
  tag scope: CWS_Safety_Limit=global, CWS_Safety_lvl=global, S5=global
  wires:
  aTemp/1 -> Bus Creator/2  "aTemp_S5"
  aPres_S4/1 -> Bus Creator/1  "aPres_S5"
  SEntropy/1 -> Bus Creator/9  "SEntropy_S5"
  MixSEnthaply/1 -> Bus Creator/6  "MixSEnthalpy_S5"
  MixDensity/1 -> Bus Creator/7  "MixDensity_S5"
  mFraction/1 -> Bus Creator/5  "mFraction_S5"
  mFlow/1 -> Bus Creator/3  "mFlow_S5"
  relHum/1 -> Bus Creator/4  "relHum_S5"
  SHeat/1 -> Bus Creator/8  "SHeat_S5"
  Bus Creator/1 -> [S5]
  relHum1/1 -> [CWS_Safety_Limit]  "SpeHum_S5"
  relHum2/1 -> [CWS_Safety_lvl]  "TGA_S5"
  connections:
  Conn2/RConn1 -- Mass & Energy Flow Rate Sensor (MA)/LConn1
  Humidity & Trace Gas Sensor (MA)1/RConn1 -- relHum/LConn1
  MixSEnthaply/LConn1 -- Thermodynamic Properties Sensor (MA)/RConn1
  MixDensity/LConn1 -- Thermodynamic Properties Sensor (MA)/RConn2
  SHeat/LConn1 -- Thermodynamic Properties Sensor (MA)/RConn4
  aTemp/LConn1 -- Pressure & Temperature Sensor (MA)/RConn3
  SEntropy/LConn1 -- Thermodynamic Properties Sensor (MA)/RConn3
  Conn1/RConn1 -- Humidity & Trace Gas Sensor (MA)2/LConn1 -- Mass & Energy Flow Rate Sensor (MA)/RConn1 -- Thermodynamic Properties Sensor (MA)/LConn1 -- Pressure & Temperature Sensor (MA)/LConn1 -- Humidity & Trace Gas Sensor (MA)1/LConn1
  mFlow/LConn1 -- Mass & Energy Flow Rate Sensor (MA)/RConn2
  Pressure & Temperature Sensor (MA)/RConn2 -- aPres_S4/LConn1
  Humidity & Trace Gas Sensor (MA)1/RConn2 -- mFraction/LConn1
  Pressure & Temperature Sensor (MA)/RConn1 -- Absolute Reference (MA)/LConn1
  Humidity & Trace Gas Sensor (MA)2/RConn1 -- relHum1/LConn1
  Humidity & Trace Gas Sensor (MA)2/RConn2 -- relHum2/LConn1

== system H175_Stage_01_Anode_Cathode/Plant Model H175-Cathode-S1/S6 ==
  Absolute Reference (MA) : fl_lib/Moist Air/Elements/Absolute Reference (MA)
  Bus Creator : BusCreator  Inputs=9
  Humidity & Trace Gas Sensor (MA)1 : fl_lib/Moist Air/Sensors/Humidity & Trace Gas Sensor (MA)  moisture_on=true  moisture_spec=foundation.enum.moisture_spec.relative_humidity  trace_gas_on=true  trace_gas_spec=foundation.enum.trace_gas_spec.mass_fraction
      settings: InternalSimscapePortConfiguration="{\"Bottom\":[],\"Left\":[{\"id\":\"A\",\"label\":\"A\",\"type\":\"foundation.moist_air.moist_air\"}],\"Right\":[{\"id\":\"W\",\"label\":\"W\",\"type\":\"output\"},{\"id\":\"G\",\"label\":\"G\",\"type\":\"output\"}],\"Top\":[]}"
  Mass & Energy Flow Rate Sensor (MA) : fl_lib/Moist Air/Sensors/Flow Rate Sensor (MA)  mass_flow_measure=true  volumetric_flow_measure=false  volumetric_flow_conditions=foundation.enum.volumetric_flow_conditions.actual  p_std=0.101325 MPa  T_std=20 degC  RH_std=0.65  energy_flow_measure=true  vapor_flow_measure=true  gas_flow_measure=true
      settings: InternalSimscapePortConfiguration="{\"Bottom\":[{\"id\":\"PHI\",\"label\":\"φ\",\"type\":\"output\"}],\"Left\":[{\"id\":\"A\",\"label\":\"A\",\"type\":\"foundation.moist_air.moist_air\"},{\"id\":\"Mw\",\"label\":\"Mw\",\"type\":\"output\"},{\"id\":\"Mg\",\"label\":\"Mg\",\"type\":\"output\"}],\"Right\":[{\"id\":\"B\",\"label\":\"B\",\"type\":\"foundation.moist_air.moist_air\"},{\"id\":\"M\",\"label\":\"M\",\"type\":\"output\"}],\"Top\":[]}"
  MixDensity : nesl_utility/PS-Simulink Converter  PhysicalDomain=network_engine_domain  SubClassName=ps_output  LeftPortType=input  RightPortType=output  PseudoPeriodic=off  Frequencies=[]  VectorFormat=inherit  Unit=inherit  AffineConversion=off
  MixSEnthaply : nesl_utility/PS-Simulink Converter  PhysicalDomain=network_engine_domain  SubClassName=ps_output  LeftPortType=input  RightPortType=output  PseudoPeriodic=off  Frequencies=[]  VectorFormat=inherit  Unit=inherit  AffineConversion=off
  Pressure & Temperature Sensor (MA) : fl_lib/Moist Air/Sensors/Pressure & Temperature Sensor (MA)  reference=foundation.enum.MeasurementReference.difference  pressure=true  pressure_spec=foundation.enum.PressureMeasementSpec.Absolute  temperature=true
      settings: InternalSimscapePortConfiguration="{\"Bottom\":[{\"id\":\"T\",\"label\":\"T\",\"type\":\"output\"}],\"Left\":[{\"id\":\"A\",\"label\":\"A\",\"type\":\"foundation.moist_air.moist_air\"}],\"Right\":[{\"id\":\"B\",\"label\":\"B\",\"type\":\"foundation.moist_air.moist_air\"},{\"id\":\"P\",\"label\":\"P\",\"type\":\"output\"}],\"Top\":[]}"
  SEntropy : nesl_utility/PS-Simulink Converter  PhysicalDomain=network_engine_domain  SubClassName=ps_output  LeftPortType=input  RightPortType=output  PseudoPeriodic=off  Frequencies=[]  VectorFormat=inherit  Unit=inherit  AffineConversion=off
  SHeat : nesl_utility/PS-Simulink Converter  PhysicalDomain=network_engine_domain  SubClassName=ps_output  LeftPortType=input  RightPortType=output  PseudoPeriodic=off  Frequencies=[]  VectorFormat=inherit  Unit=inherit  AffineConversion=off
  Thermodynamic Properties Sensor (MA) : fl_lib/Moist Air/Sensors/Thermodynamic Properties Sensor (MA)  measurement_mass_spec=foundation.enum.measurement_mass_spec.mixture  enthalpy=true  density=true  specific_heat=true  entropy=true
      settings: InternalSimscapePortConfiguration="{\"Bottom\":[{\"id\":\"CP\",\"label\":\"cp\",\"type\":\"output\"},{\"id\":\"S\",\"label\":\"s\",\"type\":\"output\"}],\"Left\":[{\"id\":\"A\",\"label\":\"A\",\"type\":\"foundation.moist_air.moist_air\"}],\"Right\":[{\"id\":\"H\",\"label\":\"h\",\"type\":\"output\"},{\"id\":\"RHO\",\"label\":\"ρ\",\"type\":\"output\"}],\"Top\":[]}"
  aPres_S4 : nesl_utility/PS-Simulink Converter  PhysicalDomain=network_engine_domain  SubClassName=ps_output  LeftPortType=input  RightPortType=output  PseudoPeriodic=off  Frequencies=[]  VectorFormat=inherit  Unit=inherit  AffineConversion=off
  aTemp : nesl_utility/PS-Simulink Converter  PhysicalDomain=network_engine_domain  SubClassName=ps_output  LeftPortType=input  RightPortType=output  PseudoPeriodic=off  Frequencies=[]  VectorFormat=inherit  Unit=inherit  AffineConversion=off
  mFlow : nesl_utility/PS-Simulink Converter  PhysicalDomain=network_engine_domain  SubClassName=ps_output  LeftPortType=input  RightPortType=output  PseudoPeriodic=off  Frequencies=[]  VectorFormat=inherit  Unit=inherit  AffineConversion=off
  mFraction : nesl_utility/PS-Simulink Converter  PhysicalDomain=network_engine_domain  SubClassName=ps_output  LeftPortType=input  RightPortType=output  PseudoPeriodic=off  Frequencies=[]  VectorFormat=inherit  Unit=inherit  AffineConversion=off
  relHum : nesl_utility/PS-Simulink Converter  PhysicalDomain=network_engine_domain  SubClassName=ps_output  LeftPortType=input  RightPortType=output  PseudoPeriodic=off  Frequencies=[]  VectorFormat=inherit  Unit=inherit  AffineConversion=off
  Conn1 : PMIOPort  Side=Left
  Conn2 : PMIOPort  Port=2  Side=Right
  tag scope: S6=global
  wires:
  SHeat/1 -> Bus Creator/8  "SHeat_S6"
  relHum/1 -> Bus Creator/4  "relHum_S6"
  mFlow/1 -> Bus Creator/3  "mFlow_S6"
  mFraction/1 -> Bus Creator/5  "mFraction_S6"
  MixDensity/1 -> Bus Creator/7  "MixDensity_S6"
  MixSEnthaply/1 -> Bus Creator/6  "MixSEnthalpy_S6"
  SEntropy/1 -> Bus Creator/9  "SEntropy_S6"
  aPres_S4/1 -> Bus Creator/1  "aPres_S6"
  aTemp/1 -> Bus Creator/2  "aTemp_S6"
  Bus Creator/1 -> [S6]
  connections:
  Humidity & Trace Gas Sensor (MA)1/RConn2 -- mFraction/LConn1
  Pressure & Temperature Sensor (MA)/RConn2 -- aPres_S4/LConn1
  mFlow/LConn1 -- Mass & Energy Flow Rate Sensor (MA)/RConn2
  Conn2/RConn1 -- Mass & Energy Flow Rate Sensor (MA)/LConn1
  SEntropy/LConn1 -- Thermodynamic Properties Sensor (MA)/RConn3
  aTemp/LConn1 -- Pressure & Temperature Sensor (MA)/RConn3
  SHeat/LConn1 -- Thermodynamic Properties Sensor (MA)/RConn4
  MixDensity/LConn1 -- Thermodynamic Properties Sensor (MA)/RConn2
  MixSEnthaply/LConn1 -- Thermodynamic Properties Sensor (MA)/RConn1
  Humidity & Trace Gas Sensor (MA)1/RConn1 -- relHum/LConn1
  Mass & Energy Flow Rate Sensor (MA)/RConn1 -- Conn1/RConn1 -- Pressure & Temperature Sensor (MA)/LConn1 -- Thermodynamic Properties Sensor (MA)/LConn1 -- Humidity & Trace Gas Sensor (MA)1/LConn1
  Absolute Reference (MA)/LConn1 -- Pressure & Temperature Sensor (MA)/RConn1
